simulink model "servoFiltro"  (R2024a)
settings: Solver=VariableStepAuto  StartTime=0.0  StopTime=50.0  RelTol=1e-3
libraries: simulink x1
settings Model: Creator=Ricky  LastModifiedBy=Ricky

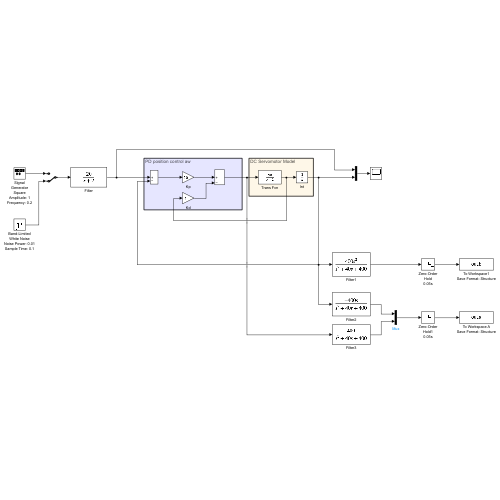
[thumbnail: Simulink's stored preview of the top-level diagram]
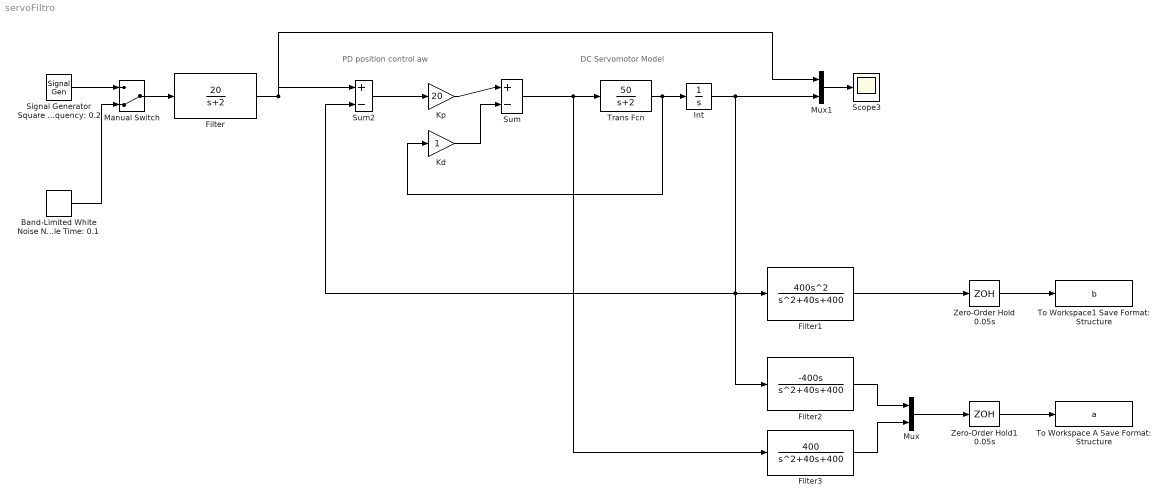
== system servoFiltro ==
  note: PD position control aw
  note: DC Servomotor Model
  Band-Limited White Noise Noise Power: 0.01 Sample Time: 0.1 : simulink/Sources/Band-Limited White Noise  Cov=[0.01]  Ts=0.1  seed=[23341]
  Filter : TransferFcn  Numerator=[20]  Denominator=[1 2]
  Filter1 : TransferFcn  Numerator=[400 0 0]  Denominator=[1 40 400]
  Filter2 : TransferFcn  Numerator=[-400 0]  Denominator=[1 40 400]
  Filter3 : TransferFcn  Numerator=[400]  Denominator=[1 40 400]
  Int : Integrator
  Kd : Gain
  Kp : Gain  Gain=20
  Manual Switch : ManualSwitch  CurrentSetting=0
  Mux : Mux  Inputs=2
  Mux1 : Mux  Inputs=2
  Scope3 : Scope
  Signal Generator Square Amplitude: 1 Frequency: 0.2 : SignalGenerator  WaveForm=square  Frequency=0.2  Units=rad/sec
  Sum : Sum  Inputs=|+-
  Sum2 : Sum  Inputs=|+-
  To Workspace A Save Format: Structure : ToWorkspace  VariableName=a  SaveFormat=Structure  SampleTime=-1
  To Workspace1 Save Format: Structure : ToWorkspace  VariableName=b  SaveFormat=Structure  SampleTime=-1
  Trans Fcn : TransferFcn  Numerator=[50]  Denominator=[1 2]
  Zero-Order Hold 0.05s : ZeroOrderHold  SampleTime=0.05
  Zero-Order Hold1 0.05s : ZeroOrderHold  SampleTime=0.05
  wires:
  Int/1 -> Sum2/2, Filter2/1, Filter1/1, Mux1/2
  Kd/1 -> Sum/2
  Sum/1 -> Filter3/1, Trans Fcn/1
  Trans Fcn/1 -> Kd/1, Int/1
  Mux1/1 -> Scope3/1
  Kp/1 -> Sum/1
  Sum2/1 -> Kp/1
  Filter/1 -> Sum2/1, Mux1/1
  Manual Switch/1 -> Filter/1
  Signal Generator Square Amplitude: 1 Frequency: 0.2/1 -> Manual Switch/1
  Band-Limited White Noise Noise Power: 0.01 Sample Time: 0.1/1 -> Manual Switch/2
  Mux/1 -> Zero-Order Hold1 0.05s/1
  Filter3/1 -> Mux/2
  Filter2/1 -> Mux/1
  Zero-Order Hold1 0.05s/1 -> To Workspace A Save Format: Structure/1
  Filter1/1 -> Zero-Order Hold 0.05s/1
  Zero-Order Hold 0.05s/1 -> To Workspace1 Save Format: Structure/1
